simulink model "main_sim"  (Simulink 7.2)
settings: Solver=ode2  SolverMode=SingleTasking  StartTime=0.0  StopTime=tsim_max  FixedStep=dtsim  RelTol=1e-3
StopFcn:
  | %mkplt
undefined symbols (not defined in the file): aero_surf_qbar_off, aero_surf_qbar_on, assertion_time, att_type, att_type_numbers, bb_ellipsoid, bb_params, compute_all_rate_cols, compute_all_vel_cols, constants, cosA, DiscIntNeverNeededParam, dtsim, E_rwy, eow_boundary, full_surf_llim, full_surf_ulim, gain_set, gain_var_struct, MACH, MACH_att_fb, MACH_gain_mat, MACH_mass_IC, MACH_pos_IC, MACH_pqr_Bmat_IC, MACH_pqr_IC, MACH_pqr_u_IC, MACH_quat_IC, MACH_throttle_IC, MACH_U_nom_IC, MACH_vel_Bmat_IC, MACH_vel_cvdnom_IC, MACH_vel_IC, MACH_vel_uold_IC, max_LOS_rate, modes, N_rwy, pos, rcs_cvddes_thresh, reset_camcmd_on_entry, sinA, target_pos_IC, target_range_blind, target_range_detect, target_range_homing, target_vel_IC, trac_params, u_llim, u_ulim, use_auto_att_type, use_eow_as_iv, use_nav, use_pos_fltpath_lim, use_throt_estimate, use_variable_mass, use_wind_est, vel, vel_cmd_ramp_time, x_trac_IC
libraries: simulink x32, mach_lib x26, utility_lib x24, model_lib x15, simulink_need_slupdate x8, models x6
(part 4 of 5)

== system main_sim/claw_main/input processing/set control parameters/accel submode setup ==
  signal_bus : Inport  OutDataType=sfix(16)  OutScaling=2^0
  Bus Selector1 : BusSelector  OutputSignals=mode_sw.enable_homing_sw,mode_sw.accel_submode,mode_sw.CLAW_mode
  Constant1 : Constant  Value=3  OutDataType=sfix(16)  OutScaling=2^0
  Constant2 : Constant  Value=0  OutDataType=sfix(16)  OutScaling=2^0
  Merge1 : Merge  Inputs=3  InitialOutput=zeros(3,1)
  Merge2 : Merge  Inputs=3  InitialOutput=zeros(3,1)
  NED_dd/vchigam_dot : Subsystem  TreatAsAtomicUnit=on
  Switch : Switch  Threshold=0.5
  Switch Case : SwitchCase  CaseConditions={[1 2],3}
  Switch1 : Switch  Threshold=0.5  InputSameDT=on
  homing : Subsystem  TreatAsAtomicUnit=on
  normal vel desdyn : Subsystem  TreatAsAtomicUnit=on
  accel_cmd_sw : Outport  OutDataType=sfix(16)  OutScaling=2^0
  accel_cmd : Outport  Port=2  OutDataType=sfix(16)  OutScaling=2^0
  wires:
  Constant1/1 -> Switch/1
  Bus Selector1/1 -> Switch/2  "<enable_homing_sw>"
  Bus Selector1/2 -> Switch/3  "<accel_submode>"
  Switch/1 -> Switch1/1
  Switch1/1 -> Switch Case/1, NED_dd/vchigam_dot/1(case)
  Switch Case/1 -> NED_dd/vchigam_dot/Action
  Switch Case/2 -> homing/Action
  Switch Case/3 -> normal vel desdyn/Action
  Merge1/1 -> accel_cmd/1
  Merge2/1 -> accel_cmd_sw/1
  NED_dd/vchigam_dot/1(accel_cmd_sw) -> Merge2/1
  normal vel desdyn/2(accel_cmd) -> Merge1/3
  NED_dd/vchigam_dot/2(accel_cmd) -> Merge1/1
  homing/2(accel_cmd) -> Merge1/2
  homing/1(accel_cmd_sw) -> Merge2/2
  normal vel desdyn/1(accel_cmd_sw) -> Merge2/3
  Bus Selector1/3 -> Switch1/2  "<CLAW_mode>"
  Constant2/1 -> Switch1/3
  signal_bus/1 -> Bus Selector1/1, NED_dd/vchigam_dot/2(signal_bus), homing/1(signal_bus)

== system main_sim/claw_main/input processing/set control parameters/modify MACH_att_Kf ==
  gain_bus_in : Inport  OutDataType=sfix(16)  OutScaling=2^0
  signal_bus : Inport  Port=2  OutDataType=sfix(16)  OutScaling=2^0
  Bus Assignment : BusAssignment  AssignedSignals=MACH_att_Kf
  Bus Selector : BusSelector  OutputSignals=mode_sw.att_type
  Bus Selector1 : BusSelector  OutputSignals=MACH_att_Kf
  Compare To Constant : simulink/Logic and Bit Operations/Compare To Constant  SystemSampleTime=-1  relop=>=  const=att_type.mba_bank  LogicOutDataTypeMode=boolean  ZeroCross=off
  Constant : Constant  Value=MACH_att_fb  OutDataType=sfix(16)  OutScaling=2^0
  Logical Operator : Logic  AllPortsSameDT=off
  Logical Operator1 : Logic  Operator=OR  AllPortsSameDT=off  OutDataTypeMode=boolean  OutDataTypeStr=boolean
  Logical Operator2 : Logic  Operator=NOT  AllPortsSameDT=off  OutDataTypeMode=boolean  OutDataTypeStr=boolean
  Logical Operator3 : Logic  AllPortsSameDT=off  OutDataTypeMode=boolean  OutDataTypeStr=boolean
  gain_bus : Outport  OutDataType=sfix(16)  OutScaling=2^0
  wires:
  Bus Selector1/1 -> Logical Operator/1  "<MACH_att_Kf>"
  Constant/1 -> Logical Operator2/1, Logical Operator3/1
  Logical Operator2/1 -> Logical Operator1/1
  gain_bus_in/1 -> Bus Assignment/1, Bus Selector1/1
  signal_bus/1 -> Bus Selector/1
  Bus Selector/1 -> Compare To Constant/1  "<att_type>"
  Logical Operator3/1 -> Logical Operator1/2
  Compare To Constant/1 -> Logical Operator3/2
  Logical Operator1/1 -> Logical Operator/2
  Logical Operator/1 -> Bus Assignment/2
  Bus Assignment/1 -> gain_bus/1

== system main_sim/claw_main/input processing/set control parameters/select gains ==
  note: Note: Current variable gain structure will use gain_set = 1
      | if it exists, when enable_bb is true, otherwise gain_set = 0
      | (which is the global or selected default)
  enable_bb : Inport  OutDataType=sfix(16)  OutScaling=2^0
  gain_set_in : Inport  Port=2  OutDataType=sfix(16)  OutScaling=2^0
  Constant2 : Constant  Value=MACH_gain_mat  OutDataType=sfix(16)  OutScaling=2^0
  MinMax : MinMax  Inputs=2  OutDataType=sfix(16)  OutScaling=2^0
  Product : Product  Inputs=*/  OutDataType=sfix(16)  OutScaling=2^0  RndMeth=Zero
  Reshape : Reshape
  Switch : Switch
  Width1 : Width
  Width2 : Width
  mux to bus : Subsystem  mask{var_struct=gain_var_struct}
      mask prompts: var_struct "var struct"
      mask init:
      | if(~isstruct(var_struct) || length(var_struct) == 0 || ~isfield(var_struct,'name') || ~isfield(var_struct,'size'))
      |     error('var struct must be at least size 1, and must have the ''name'' and ''size'' fields defined.');
      | end
      | 
      | var_name = {var_struct.name};
      | var_size = prod(vertcat(var_struct.size),2);
      | nvar = length(var_name);
      | 
      | % remove old lines
      | nvar_old = length(get_param([gcb '/Demux'],'Outputs'));
      | for i = 1:nvar_old
      |     try
      |         delete_line(gcb,['Demux/' num2str(i)] ,['Bus Creator/' num2str(i)])
      |     end
      | end
      | 
      | set_param([gcb '/Demux'],'Outputs',mat2str(var_size));
      | set_param([gcb '/Bus Creator'],'Inputs',num2str(nvar));
      | port_handle = getfield(get_param([gcb '/Demux'],'PortHandles'),'Outport');
      | for i = 1:nvar
      |     try
      |         add_line(gcb,['Demux/' num2str(i)] ,['Bus Creator/' num2str(i)])
      |     end
      |     set(port_handle(i),'Name',var_name{i});
      | end
  select gain set : Selector  NumberOfDimensions=2  IndexMode=Zero-based  InputPortWidth=3  IndexOptions=Index vector (port),Select all  Indices=gain_set,-1  OutputSizes=1
  gain_set : Outport  OutDataType=sfix(16)  OutScaling=2^0
  gain_bus : Outport  Port=2  OutDataType=sfix(16)  OutScaling=2^0
  wires:
  Constant2/1 -> select gain set/1, Width2/1
  select gain set/1 -> Reshape/1
  Reshape/1 -> mux to bus/1(mux_in), Width1/1
  MinMax/1 -> gain_set/1, select gain set/2
  enable_bb/1 -> Switch/3
  mux to bus/1(bus_out) -> gain_bus/1
  Width2/1 -> Product/1
  Width1/1 -> Product/2
  gain_set_in/1 -> Switch/1, Switch/2
  Switch/1 -> MinMax/1
  Product/1 -> MinMax/2

== system main_sim/claw_main/input processing/set control parameters/set att desdyn params ==
  gain_bus : Inport  OutDataType=sfix(16)  OutScaling=2^0
  Bus Creator : BusCreator  Inputs=7
  Bus Selector : BusSelector  OutputSignals=MACH_att_Kb,MACH_att_Ki,MACH_att_Kaw,MACH_att_Kf
  Constant1 : Constant  Value=zeros(1,4)  OutDataType=sfix(16)  OutScaling=2^0
  Constant6 : Constant  Value=MACH_quat_IC  OutDataType=sfix(16)  OutScaling=2^0
  Signal Specification : SignalSpecification  OutDataType=sfix(16)  OutScaling=2^0
  Signal Specification1 : SignalSpecification  OutDataType=sfix(16)  OutScaling=2^0
  Signal Specification2 : SignalSpecification  OutDataType=sfix(16)  OutScaling=2^0
  compute dependent gains : mach_lib/compute dependent gains  SystemSampleTime=-1
  params : Outport  OutDataType=sfix(16)  OutScaling=2^0
  wires:
  compute dependent gains/4 -> Bus Creator/6  "x0"
  Bus Selector/3 -> compute dependent gains/3  "<MACH_att_Kaw>"
  compute dependent gains/2 -> Bus Creator/4  "ki_trim"
  compute dependent gains/1 -> Bus Creator/3  "kc"
  Bus Creator/1 -> params/1
  Bus Selector/1 -> Signal Specification/1  "<MACH_att_Kb>"
  Bus Selector/2 -> Signal Specification1/1  "<MACH_att_Ki>"
  compute dependent gains/3 -> Bus Creator/5  "kaw"
  Bus Selector/4 -> Signal Specification2/1, compute dependent gains/4  "<MACH_att_Kf>"
  gain_bus/1 -> Bus Selector/1
  Signal Specification/1 -> Bus Creator/1, compute dependent gains/2  "kb"
  Signal Specification1/1 -> Bus Creator/2, compute dependent gains/1  "ki"
  Signal Specification2/1 -> Bus Creator/7  "kf"
  Constant6/1 -> compute dependent gains/5
  Constant1/1 -> compute dependent gains/6

== system main_sim/claw_main/input processing/set control parameters/set pos desdyn params ==
  gain_bus : Inport  OutDataType=sfix(16)  OutScaling=2^0
  Bus Creator : BusCreator  Inputs=7
  Bus Selector : BusSelector  OutputSignals=MACH_pos_Kb,MACH_pos_Ki,MACH_pos_Kaw,MACH_pos_Kf
  Constant3 : Constant  Value=MACH_vel_IC  OutDataType=sfix(16)  OutScaling=2^0
  Constant6 : Constant  Value=MACH_pos_IC  OutDataType=sfix(16)  OutScaling=2^0
  Signal Specification : SignalSpecification  OutDataType=sfix(16)  OutScaling=2^0
  Signal Specification1 : SignalSpecification  OutDataType=sfix(16)  OutScaling=2^0
  Signal Specification2 : SignalSpecification  OutDataType=sfix(16)  OutScaling=2^0
  compute dependent gains : mach_lib/compute dependent gains  SystemSampleTime=-1
  params : Outport  OutDataType=sfix(16)  OutScaling=2^0
  wires:
  Bus Selector/3 -> compute dependent gains/3  "<MACH_pos_Kaw>"
  compute dependent gains/2 -> Bus Creator/4  "ki_trim"
  compute dependent gains/1 -> Bus Creator/3  "kc"
  Bus Creator/1 -> params/1
  Bus Selector/1 -> Signal Specification/1  "<MACH_pos_Kb>"
  Bus Selector/2 -> Signal Specification1/1  "<MACH_pos_Ki>"
  compute dependent gains/3 -> Bus Creator/5  "kaw"
  Bus Selector/4 -> Signal Specification2/1, compute dependent gains/4  "<MACH_pos_Kf>"
  compute dependent gains/4 -> Bus Creator/6  "x0"
  gain_bus/1 -> Bus Selector/1
  Signal Specification/1 -> Bus Creator/1, compute dependent gains/2  "kb"
  Signal Specification1/1 -> compute dependent gains/1, Bus Creator/2  "ki"
  Signal Specification2/1 -> Bus Creator/7  "kf"
  Constant6/1 -> compute dependent gains/5
  Constant3/1 -> compute dependent gains/6

== system main_sim/claw_main/input processing/set control parameters/set rate desdyn params ==
  gain_bus : Inport  OutDataType=sfix(16)  OutScaling=2^0
  Bus Creator : BusCreator  Inputs=7
  Bus Selector : BusSelector  OutputSignals=MACH_pqr_Kb,MACH_pqr_Ki,MACH_pqr_Kaw,MACH_pqr_Kf
  Constant1 : Constant  Value=zeros(1,3)  OutDataType=sfix(16)  OutScaling=2^0
  Constant6 : Constant  Value=MACH_pqr_IC  OutDataType=sfix(16)  OutScaling=2^0
  Signal Specification : SignalSpecification  OutDataType=sfix(16)  OutScaling=2^0
  Signal Specification1 : SignalSpecification  OutDataType=sfix(16)  OutScaling=2^0
  Signal Specification2 : SignalSpecification  OutDataType=sfix(16)  OutScaling=2^0
  compute dependent gains : mach_lib/compute dependent gains  SystemSampleTime=-1
  params : Outport  OutDataType=sfix(16)  OutScaling=2^0
  wires:
  Bus Selector/4 -> Signal Specification2/1  "<MACH_pqr_Kf>"
  compute dependent gains/3 -> Bus Creator/5  "kaw"
  Signal Specification1/1 -> compute dependent gains/1, Bus Creator/2  "ki"
  Signal Specification/1 -> compute dependent gains/2, Bus Creator/1  "kb"
  Bus Creator/1 -> params/1
  compute dependent gains/1 -> Bus Creator/3  "kc"
  compute dependent gains/2 -> Bus Creator/4  "ki_trim"
  Bus Selector/3 -> compute dependent gains/3  "<MACH_pqr_Kaw>"
  compute dependent gains/4 -> Bus Creator/6  "x0"
  gain_bus/1 -> Bus Selector/1
  Bus Selector/1 -> Signal Specification/1  "<MACH_pqr_Kb>"
  Bus Selector/2 -> Signal Specification1/1  "<MACH_pqr_Ki>"
  Signal Specification2/1 -> Bus Creator/7, compute dependent gains/4  "kf"
  Constant6/1 -> compute dependent gains/5
  Constant1/1 -> compute dependent gains/6

== system main_sim/claw_main/input processing/set control parameters/set rate di params ==
  full_surf : Inport  OutDataType=sfix(16)  OutScaling=2^0
  aero_env_est : Inport  Port=2  OutDataType=sfix(16)  OutScaling=2^0
  Bus Creator1 : BusCreator  Inputs=7
  Bus Selector1 : BusSelector  OutputSignals=full_surf_ulim,full_surf_llim
  Bus Selector2 : BusSelector  OutputSignals=full_surf_urlim,full_surf_lrlim
  Bus Selector3 : BusSelector  OutputSignals=qbar
  Constant5 : Constant  Value=MACH.pqr_wght_cv  OutDataType=sfix(16)  OutScaling=2^0
  Relay : Relay  OnSwitchValue=aero_surf_qbar_on  OffSwitchValue=aero_surf_qbar_off  OnOutputValue=0  OffOutputValue=1  OutDataType=sfix(16)  OutScaling=2^0
  Selector{1..2,5..6} (4 alike) : Selector  InputPortWidth=MACH.num_u  IndexOptions=Index vector (dialog)  Indices=MACH.pqr_u_idx  OutputSizes=1
  fix aero surfs when low qbar : Subsystem
  limit schedule : model_lib/no limit schedule  SystemSampleTime=-1
  select u_pref : Subsystem
  rate_params : Outport  OutDataType=sfix(16)  OutScaling=2^0
  wires:
  select u_pref/2(wght_u_pref) -> Bus Creator1/6  "wght_u_pref"
  select u_pref/1(u_pref) -> Bus Creator1/5, fix aero surfs when low qbar/4(pqr_u_pref)  "u_pref"
  Bus Creator1/1 -> rate_params/1
  full_surf/1 -> Bus Selector1/1, Bus Selector2/1, select u_pref/3(full_surf)
  Selector6/1 -> limit schedule/2
  Bus Selector1/1 -> Selector5/1  "<full_surf_ulim>"
  Bus Selector1/2 -> Selector6/1  "<full_surf_llim>"
  Selector5/1 -> limit schedule/1
  aero_env_est/1 -> select u_pref/2(aero_env_est), limit schedule/3, Bus Selector3/1
  Selector1/1 -> Bus Creator1/1  "u_urlim"
  Selector2/1 -> Bus Creator1/2  "u_lrlim"
  fix aero surfs when low qbar/1(pqr_u_ulim) -> Bus Creator1/3  "u_ulim"
  fix aero surfs when low qbar/2(pqr_u_llim) -> Bus Creator1/4  "u_llim"
  limit schedule/1 -> fix aero surfs when low qbar/1(pqr_u_ulim_in)
  limit schedule/2 -> fix aero surfs when low qbar/2(pqr_u_llim_in)
  Bus Selector2/1 -> Selector1/1  "<full_surf_urlim>"
  Bus Selector2/2 -> Selector2/1  "<full_surf_lrlim>"
  Constant5/1 -> Bus Creator1/7  "wght_cv"
  Bus Selector3/1 -> Relay/1  "<qbar>"
  Relay/1 -> fix aero surfs when low qbar/3(low_qbar), select u_pref/1(low_qbar)

== system main_sim/claw_main/input processing/set control parameters/set vel desdyn params ==
  gain_bus : Inport  OutDataType=sfix(16)  OutScaling=2^0
  Bus Creator : BusCreator  Inputs=7
  Bus Selector : BusSelector  OutputSignals=MACH_vel_Kb,MACH_vel_Ki,MACH_vel_Kaw,MACH_vel_Kf
  Constant1 : Constant  Value=MACH_vel_cvdnom_IC  OutDataType=sfix(16)  OutScaling=2^0
  Constant6 : Constant  Value=MACH_vel_IC  OutDataType=sfix(16)  OutScaling=2^0
  Signal Specification : SignalSpecification  OutDataType=sfix(16)  OutScaling=2^0
  Signal Specification1 : SignalSpecification  OutDataType=sfix(16)  OutScaling=2^0
  Signal Specification2 : SignalSpecification  OutDataType=sfix(16)  OutScaling=2^0
  compute dependent gains : mach_lib/compute dependent gains  SystemSampleTime=-1
  params : Outport  OutDataType=sfix(16)  OutScaling=2^0
  wires:
  Bus Selector/4 -> Signal Specification2/1, compute dependent gains/4  "<MACH_vel_Kf>"
  compute dependent gains/3 -> Bus Creator/5  "kaw"
  Bus Selector/2 -> Signal Specification1/1  "<MACH_vel_Ki>"
  Bus Selector/1 -> Signal Specification/1  "<MACH_vel_Kb>"
  Bus Creator/1 -> params/1
  compute dependent gains/1 -> Bus Creator/3  "kc"
  compute dependent gains/2 -> Bus Creator/4  "ki_trim"
  Bus Selector/3 -> compute dependent gains/3  "<MACH_vel_Kaw>"
  gain_bus/1 -> Bus Selector/1
  Signal Specification/1 -> Bus Creator/1, compute dependent gains/2  "kb"
  Signal Specification1/1 -> compute dependent gains/1, Bus Creator/2  "ki"
  Signal Specification2/1 -> Bus Creator/7  "kf"
  compute dependent gains/4 -> Bus Creator/6  "x0"
  Constant6/1 -> compute dependent gains/5
  Constant1/1 -> compute dependent gains/6

== system main_sim/claw_main/rate_loops/B matrix comp/cvd_def_nom ==
  x : Inport  OutDataType=sfix(16)  OutScaling=2^0
  u : Inport  Port=2  OutDataType=sfix(16)  OutScaling=2^0
  xdot : Inport  Port=3  OutDataType=sfix(16)  OutScaling=2^0
  Selector : Selector  InputPortWidth=MACH.num_x  IndexOptions=Index vector (dialog)  Indices=MACH.pqr_idx  OutputSizes=1
  Terminator : Terminator
  Terminator1 : Terminator
  cvd : Outport  OutDataType=sfix(16)  OutScaling=2^0
  wires:
  xdot/1 -> Selector/1
  Selector/1 -> cvd/1
  u/1 -> Terminator/1
  x/1 -> Terminator1/1

== system main_sim/claw_main/rate_loops/B matrix comp/cvd_def_pert ==
  x : Inport  OutDataType=sfix(16)  OutScaling=2^0
  u : Inport  Port=2  OutDataType=sfix(16)  OutScaling=2^0
  xdot : Inport  Port=3  OutDataType=sfix(16)  OutScaling=2^0
  Selector : Selector  InputPortWidth=MACH.num_x  IndexOptions=Index vector (dialog)  Indices=MACH.pqr_idx  OutputSizes=1
  Terminator : Terminator
  Terminator1 : Terminator
  cvd : Outport  OutDataType=sfix(16)  OutScaling=2^0
  wires:
  xdot/1 -> Selector/1
  Selector/1 -> cvd/1
  u/1 -> Terminator/1
  x/1 -> Terminator1/1

== system main_sim/claw_main/rate_loops/B matrix comp/pert insert ==
  X_nom : Inport  OutDataType=sfix(16)  OutScaling=2^0
  U_nom : Inport  Port=2  OutDataType=sfix(16)  OutScaling=2^0
  D_pert : Inport  Port=3  OutDataType=sfix(16)  OutScaling=2^0
  Assignment : Assignment  IndexOptions=Index vector (dialog)  Indices=MACH.pqr_u_idx  OutputSizes=[1 1]
  X_pert : Outport  OutDataType=sfix(16)  OutScaling=2^0
  U_pert : Outport  Port=2  OutDataType=sfix(16)  OutScaling=2^0
  wires:
  D_pert/1 -> Assignment/2
  Assignment/1 -> U_pert/1
  X_nom/1 -> X_pert/1
  U_nom/1 -> Assignment/1

== system main_sim/claw_main/rate_loops/B matrix comp/pert_comp ==
  col : Inport  OutDataType=sfix(16)  OutScaling=2^0
  d_nom : Inport  Port=2  OutDataType=sfix(16)  OutScaling=2^0
  params : Inport  Port=3  OutDataType=sfix(16)  OutScaling=2^0
  Bus Selector : BusSelector  OutputSignals=u_ulim,u_llim
  Constant2 : Constant  Value=diag(MACH.pqr_u_pert)  OutDataType=sfix(16)  OutScaling=2^0
  pick +/- pert : mach_lib/pick +//- pert  SystemSampleTime=-1  num_u=MACH.pqr_num_u
  d_pert : Outport  OutDataType=sfix(16)  OutScaling=2^0
  d_div : Outport  Port=2  OutDataType=sfix(16)  OutScaling=2^0
  wires:
  Constant2/1 -> pick +/- pert/5
  pick +/- pert/1 -> d_pert/1
  pick +/- pert/2 -> d_div/1  "scalar pert value"
  col/1 -> pick +/- pert/1
  d_nom/1 -> pick +/- pert/2
  Bus Selector/1 -> pick +/- pert/3  "<u_ulim>"
  params/1 -> Bus Selector/1
  Bus Selector/2 -> pick +/- pert/4  "<u_llim>"

== system main_sim/claw_main/rate_loops/allocation/RCS allocation ==
  Bmat : Inport  OutDataType=sfix(16)  OutScaling=2^0
  rcs_cmd_old : Inport  Port=2  OutDataType=sfix(16)  OutScaling=2^0
  cvd_des : Inport  Port=3  OutDataType=sfix(16)  OutScaling=2^0
  params : Inport  Port=4  OutDataType=sfix(16)  OutScaling=2^0
  Bus Selector : BusSelector  OutputSignals=wght_cv,u_ulim,u_llim
  Constant : Constant  Value=[1 1 1]  OutDataType=sfix(16)  OutScaling=2^0
  Constant1 : Constant  Value=MACH.pqr_rcs_use  OutDataType=sfix(16)  OutScaling=2^0
  Constant2 : Constant  Value=rcs_cvddes_thresh  OutDataType=sfix(16)  OutScaling=2^0
  Embedded MATLAB Function : Stateflow chart
  Sum5 : Sum  Inputs=+-|  OutDataType=sfix(16)  OutScaling=2^0  SaturateOnIntegerOverflow=on  InputSameDT=on  OutDataTypeStr=Inherit: Same as first input
  Terminator{,1..3} (4 alike) : Terminator
  rcs_cmd : Outport  OutDataType=sfix(16)  OutScaling=2^0
  cvd_extra : Outport  Port=2  OutDataType=sfix(16)  OutScaling=2^0
  wires:
  Embedded MATLAB Function/3(scale) -> Terminator3/1
  params/1 -> Bus Selector/1
  cvd_des/1 -> Sum5/2, Embedded MATLAB Function/5(cvd_des)
  Sum5/1 -> cvd_extra/1
  Bmat/1 -> Embedded MATLAB Function/1(Bmat)
  Embedded MATLAB Function/1(rcs_cmd) -> rcs_cmd/1
  Embedded MATLAB Function/2(minerr) -> Terminator2/1
  Embedded MATLAB Function/4(cvd_actual) -> Sum5/1
  rcs_cmd_old/1 -> Terminator/1
  Constant2/1 -> Embedded MATLAB Function/6(err_thresh)
  Bus Selector/3 -> Embedded MATLAB Function/4(llim)  "<u_llim>"
  Bus Selector/2 -> Embedded MATLAB Function/3(ulim)  "<u_ulim>"
  Constant1/1 -> Embedded MATLAB Function/7(rcs_use_in)
  Bus Selector/1 -> Terminator1/1  "<wght_cv>"
  Constant/1 -> Embedded MATLAB Function/2(wght_cv)

== system main_sim/claw_main/rate_loops/allocation/config_di ==
  cvd_nom : Inport  OutDataType=sfix(16)  OutScaling=2^0
  Bmat : Inport  Port=2  OutDataType=sfix(16)  OutScaling=2^0
  d_old : Inport  Port=3  OutDataType=sfix(16)  OutScaling=2^0
  d_nom : Inport  Port=4  OutDataType=sfix(16)  OutScaling=2^0
  cvd_des : Inport  Port=5  OutDataType=sfix(16)  OutScaling=2^0
  params : Inport  Port=6  OutDataType=sfix(16)  OutScaling=2^0
  di_smn : mach_lib/di_smn  SystemSampleTime=-1
  d_cmd : Outport  OutDataType=sfix(16)  OutScaling=2^0
  cvd_extra : Outport  Port=2  OutDataType=sfix(16)  OutScaling=2^0
  lambda : Outport  Port=3  OutDataType=sfix(16)  OutScaling=2^0
  solve_dat : Outport  Port=4  OutDataType=sfix(16)  OutScaling=2^0
  wires:
  cvd_nom/1 -> di_smn/1
  Bmat/1 -> di_smn/2
  d_old/1 -> di_smn/3
  d_nom/1 -> di_smn/4
  cvd_des/1 -> di_smn/5
  params/1 -> di_smn/6
  di_smn/1 -> d_cmd/1
  di_smn/2 -> cvd_extra/1
  di_smn/3 -> lambda/1
  di_smn/4 -> solve_dat/1

== system main_sim/claw_main/rate_loops/allocation/param select rcs ==
  params_all : Inport  OutDataType=sfix(16)  OutScaling=2^0
  Bus Creator1 : BusCreator  Inputs=7
  Bus Selector : BusSelector  OutputSignals=u_ulim,u_llim,u_urlim,u_lrlim,u_pref,wght_u_pref,wght_cv
  Selector{,1..5} (6 alike) : Selector  InputPortWidth=MACH.pqr_num_u  IndexOptions=Index vector (dialog)  Indices=idx  OutputSizes=1
  params : Outport  OutDataType=sfix(16)  OutScaling=2^0
  wires:
  Bus Creator1/1 -> params/1
  Bus Selector/6 -> Selector5/1  "<wght_u_pref>"
  Bus Selector/5 -> Selector4/1  "<u_pref>"
  Bus Selector/4 -> Selector3/1  "<u_lrlim>"
  Bus Selector/3 -> Selector2/1  "<u_urlim>"
  Bus Selector/2 -> Selector1/1  "<u_llim>"
  Bus Selector/1 -> Selector/1  "<u_ulim>"
  params_all/1 -> Bus Selector/1
  Selector3/1 -> Bus Creator1/4  "u_lrlim"
  Selector2/1 -> Bus Creator1/3  "u_urlim"
  Selector/1 -> Bus Creator1/1  "u_ulim"
  Selector1/1 -> Bus Creator1/2  "u_llim"
  Selector4/1 -> Bus Creator1/5  "u_pref"
  Selector5/1 -> Bus Creator1/6  "wght_u_pref"
  Bus Selector/7 -> Bus Creator1/7  "<wght_cv>"

== system main_sim/claw_main/rate_loops/allocation/param select smn ==
  params_all : Inport  OutDataType=sfix(16)  OutScaling=2^0
  Bus Creator1 : BusCreator  Inputs=7
  Bus Selector : BusSelector  OutputSignals=u_ulim,u_llim,u_urlim,u_lrlim,u_pref,wght_u_pref,wght_cv
  Selector{,1..5} (6 alike) : Selector  InputPortWidth=MACH.pqr_num_u  IndexOptions=Index vector (dialog)  Indices=idx  OutputSizes=1
  params : Outport  OutDataType=sfix(16)  OutScaling=2^0
  wires:
  Bus Selector/7 -> Bus Creator1/7  "<wght_cv>"
  Selector5/1 -> Bus Creator1/6  "wght_u_pref"
  Selector4/1 -> Bus Creator1/5  "u_pref"
  Selector1/1 -> Bus Creator1/2  "u_llim"
  Selector/1 -> Bus Creator1/1  "u_ulim"
  Selector2/1 -> Bus Creator1/3  "u_urlim"
  Selector3/1 -> Bus Creator1/4  "u_lrlim"
  params_all/1 -> Bus Selector/1
  Bus Selector/1 -> Selector/1  "<u_ulim>"
  Bus Selector/2 -> Selector1/1  "<u_llim>"
  Bus Selector/3 -> Selector2/1  "<u_urlim>"
  Bus Selector/4 -> Selector3/1  "<u_lrlim>"
  Bus Selector/5 -> Selector4/1  "<u_pref>"
  Bus Selector/6 -> Selector5/1  "<wght_u_pref>"
  Bus Creator1/1 -> params/1

== system main_sim/claw_main/rate_loops/select rate cmd/get direct cmd ==
  signal_bus : Inport  OutDataType=sfix(16)  OutScaling=2^0
  Bus Selector1 : BusSelector  OutputSignals=cmd_bus.autopilot_cmd,mode_sw.full_surf_cmd_sw,full_surf.full_surf_cmd
  Demux2 : Demux  Outputs=[ 3 1 ]
  Gain1 : Gain  Gain=MACH.throt_mixer  ParameterDataType=sfix(16)  ParameterScaling=2^0  OutDataType=sfix(16)  OutScaling=2^0
  Multiport Switch2 : MultiPortSwitch  Inputs=2  zeroidx=on
  Mux2 : Mux  Inputs=2
  throttle : Selector  InputPortWidth=MACH.num_u  IndexOptions=Index vector (dialog)  Indices=MACH.throttle_idx  OutputSizes=1
  direct_cmd : Outport  OutDataType=sfix(16)  OutScaling=2^0
  wires:
  Demux2/1 -> Mux2/1
  Demux2/2 -> Gain1/1
  Mux2/1 -> direct_cmd/1
  signal_bus/1 -> Bus Selector1/1
  Bus Selector1/1 -> Demux2/1  "<autopilot_cmd>"
  Bus Selector1/2 -> Multiport Switch2/1  "<full_surf_cmd_sw>"
  Gain1/1 -> Multiport Switch2/2
  Bus Selector1/3 -> throttle/1  "<full_surf_cmd>"
  throttle/1 -> Multiport Switch2/3
  Multiport Switch2/1 -> Mux2/2

== system main_sim/claw_main/state est/process sensors/compute dc_fltpath ==
  NEh_dot_fltpath : Inport  OutDataType=sfix(16)  OutScaling=2^0
  Gain : Gain  Gain=repmat([1 1 -1],3,1)  ParameterDataType=sfix(16)  ParameterScaling=2^0  OutDataType=sfix(16)  OutScaling=2^0
  Gain1 : Gain  Gain=[1 1 -1]  ParameterDataType=sfix(16)  ParameterScaling=2^0  OutDataType=sfix(16)  OutScaling=2^0
  Reshape : Reshape  OutputDimensionality=Customize  OutputDimensions=[3 3]
  Terminator : Terminator
  vec2dc : utility_lib/vec2dc  SystemSampleTime=-1
  dc_fltpath : Outport  OutDataType=sfix(16)  OutScaling=2^0
  wires:
  vec2dc/1 -> Reshape/1
  Reshape/1 -> Gain/1
  Gain1/1 -> vec2dc/1
  vec2dc/2 -> Terminator/1
  Gain/1 -> dc_fltpath/1
  NEh_dot_fltpath/1 -> Gain1/1

== system main_sim/claw_main/state est/process sensors/navigation complementary filter ==
  NEh nav : Inport  OutDataType=sfix(16)  OutScaling=2^0
  NEh dot : Inport  Port=2  OutDataType=sfix(16)  OutScaling=2^0
  Gain1 : Gain  Gain=MACH.K_velpos  ParameterDataType=sfix(16)  ParameterScaling=2^0  OutDataType=sfix(16)  OutScaling=2^0  SaturateOnIntegerOverflow=on  OutDataTypeStr=Inherit: Same as input  ParamDataTypeStr=Inherit: Same as input
  Sum1 : Sum  Inputs=|+-  OutDataType=sfix(16)  OutScaling=2^0  SaturateOnIntegerOverflow=on
  Sum2 : Sum  Inputs=++|  OutDataType=sfix(16)  OutScaling=2^0  SaturateOnIntegerOverflow=on  InputSameDT=on  OutDataTypeStr=Inherit: Same as first input
  integration1 : DiscreteIntegrator  SampleTime=-1  OutDataType=sfix(16)  OutScaling=2^0  ICPrevOutput=DiscIntNeverNeededParam  ICPrevScaledInput=DiscIntNeverNeededParam
  NEh_fil : Outport  OutDataType=sfix(16)  OutScaling=2^0
  wires:
  NEh dot/1 -> Sum2/1
  NEh nav/1 -> Sum1/1
  Gain1/1 -> Sum2/2
  Sum2/1 -> integration1/1
  integration1/1 -> NEh_fil/1, Sum1/2
  Sum1/1 -> Gain1/1

== system main_sim/claw_main/state est/process sensors/select e sign ==
  e in : Inport  OutDataType=sfix(16)  OutScaling=2^0
  e_past : Inport  Port=2  OutDataType=sfix(16)  OutScaling=2^0
  Dot Product : simulink/Math Operations/Dot Product  InputSameDT=on  OutDataType=sfix(16)  OutScaling=2^-10  DoSatur=off
  Gain : Gain  Gain=-1  ParameterDataType=sfix(16)  ParameterScaling=2^0  OutDataType=sfix(16)  OutScaling=2^0  SaturateOnIntegerOverflow=on  OutDataTypeStr=Inherit: Same as input  ParamDataTypeStr=Inherit: Same as input
  Switch : Switch  SaturateOnIntegerOverflow=on
  e out : Outport  OutDataType=sfix(16)  OutScaling=2^0
  wires:
  e_past/1 -> Dot Product/2
  Switch/1 -> e out/1
  Gain/1 -> Switch/3
  Dot Product/1 -> Switch/2
  e in/1 -> Gain/1, Switch/1, Dot Product/1

== system main_sim/claw_main/state est/process sensors/wait for valid nav ==
  latlonh : Inport  OutDataType=sfix(16)  OutScaling=2^0
  nav_ok : Inport  Port=2  OutDataType=sfix(16)  OutScaling=2^0
  Switch3 : Switch  Threshold=0.5  SaturateOnIntegerOverflow=on
  Unit Delay1 : UnitDelay  Orientation=left  SampleTime=-1
  LLh_0 : Outport  OutDataType=sfix(16)  OutScaling=2^0
  nav_valid : Outport  Port=2  OutDataType=sfix(16)  OutScaling=2^0
  wires:
  nav_ok/1 -> nav_valid/1, Switch3/2
  latlonh/1 -> Switch3/3
  Switch3/1 -> Unit Delay1/1, LLh_0/1
  Unit Delay1/1 -> Switch3/1

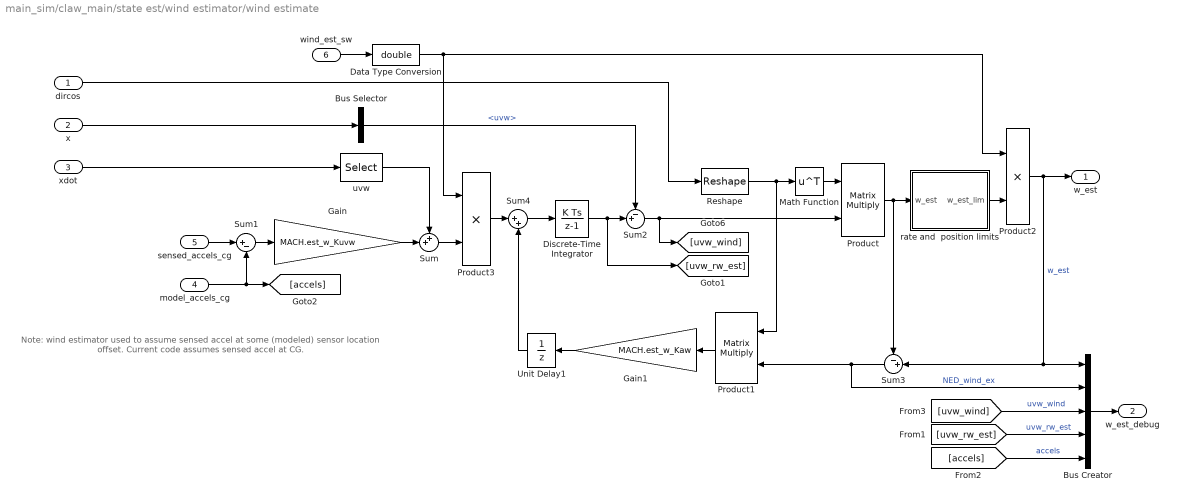
== system main_sim/claw_main/state est/wind estimator/wind estimate ==
  note: Note: wind estimator used to assume sensed accel
      | at some (modeled) sensor location offset.
      |  Current code assumes sensed accel at CG.
  dircos : Inport  OutDataType=sfix(16)  OutScaling=2^0
  x : Inport  Port=2  OutDataType=sfix(16)  OutScaling=2^0
  xdot : Inport  Port=3  OutDataType=sfix(16)  OutScaling=2^0
  model_accels_cg : Inport  Port=4  OutDataType=sfix(16)  OutScaling=2^0
  sensed_accels_cg : Inport  Port=5  OutDataType=sfix(16)  OutScaling=2^0
  wind_est_sw : Inport  Port=6  OutDataType=sfix(16)  OutScaling=2^0
  Bus Creator : BusCreator  Inputs=5
  Bus Selector : BusSelector  OutputSignals=uvw
  Data Type Conversion : DataTypeConversion  OutDataTypeMode=double  OutDataType=sfix(16)  OutScaling=2^0  OutDataTypeStr=double  SaturateOnIntegerOverflow=on  RndMeth=Zero
  Discrete-Time Integrator : DiscreteIntegrator  SampleTime=-1  OutDataType=sfix(16)  OutScaling=2^0  ICPrevOutput=DiscIntNeverNeededParam  ICPrevScaledInput=DiscIntNeverNeededParam
  Gain : Gain  Gain=MACH.est_w_Kuvw  ParameterDataType=sfix(16)  ParameterScaling=2^0  OutDataType=sfix(16)  OutScaling=2^0  SaturateOnIntegerOverflow=on  OutDataTypeStr=Inherit: Same as input  ParamDataTypeStr=Inherit: Same as input
  Gain1 : Gain  Orientation=left  Gain=MACH.est_w_Kaw  ParameterDataType=sfix(16)  ParameterScaling=2^0  OutDataType=sfix(16)  OutScaling=2^0  SaturateOnIntegerOverflow=on  OutDataTypeStr=Inherit: Same as input  ParamDataTypeStr=Inherit: Same as input
  Math Function : Math  Operator=transpose  OutDataType=sfix(16)  OutScaling=2^0  SaturateOnIntegerOverflow=on
  Product : Product  Multiplication=Matrix(*)  OutDataType=sfix(16)  OutScaling=2^0  SaturateOnIntegerOverflow=on  OutDataTypeStr=Inherit: Same as first input
  Product1 : Product  Orientation=left  Multiplication=Matrix(*)  OutDataType=sfix(16)  OutScaling=2^0  SaturateOnIntegerOverflow=on  OutDataTypeStr=Inherit: Same as first input
  Product2 : Product  OutDataType=sfix(16)  OutScaling=2^0  SaturateOnIntegerOverflow=on  OutDataTypeStr=Inherit: Same as first input
  Product3 : Product  OutDataType=sfix(16)  OutScaling=2^0  SaturateOnIntegerOverflow=on  OutDataTypeStr=Inherit: Same as first input
  Reshape : Reshape  OutputDimensionality=Customize  OutputDimensions=[3,3]
  Sum : Sum  Inputs=++|  OutDataType=sfix(16)  OutScaling=2^0  SaturateOnIntegerOverflow=on  InputSameDT=on  OutDataTypeStr=Inherit: Same as first input
  Sum1 : Sum  Inputs=|+-  OutDataType=sfix(16)  OutScaling=2^0  SaturateOnIntegerOverflow=on  InputSameDT=on  OutDataTypeStr=Inherit: Same as first input
  Sum2 : Sum  Inputs=-+|  OutDataType=sfix(16)  OutScaling=2^0  SaturateOnIntegerOverflow=on
  Sum3 : Sum  Orientation=left  Inputs=-+|  OutDataType=sfix(16)  OutScaling=2^0  SaturateOnIntegerOverflow=on
  Sum4 : Sum  Inputs=|++  OutDataType=sfix(16)  OutScaling=2^0  SaturateOnIntegerOverflow=on  InputSameDT=on  OutDataTypeStr=Inherit: Same as first input
  Unit Delay1 : UnitDelay  Orientation=left  X0=zeros(3,1)  SampleTime=-1
  rate and  position limits : Subsystem
  uvw : Selector  InputPortWidth=MACH.num_x  IndexOptions=Index vector (dialog)  Indices=MACH.uvw_idx  OutputSizes=1
  w_est : Outport  OutDataType=sfix(16)  OutScaling=2^0
  w_est_debug : Outport  Port=2  OutDataType=sfix(16)  OutScaling=2^0
  wires:
  Discrete-Time Integrator/1 -> Sum2/2, [uvw_rw_est]
  sensed_accels_cg/1 -> Sum1/1
  Sum1/1 -> Gain/1
  Sum/1 -> Product3/2
  Gain/1 -> Sum/2
  Bus Selector/1 -> Sum2/1  "<uvw>"
  dircos/1 -> Reshape/1
  Reshape/1 -> Math Function/1, Product1/1
  Product/1 -> Sum3/1, rate and  position limits/1(w_est)
  Math Function/1 -> Product/1
  Sum2/1 -> Product/2, [uvw_wind]
  Gain1/1 -> Unit Delay1/1
  xdot/1 -> uvw/1
  uvw/1 -> Sum/1
  x/1 -> Bus Selector/1
  rate and  position limits/1(w_est_lim) -> Product2/2
  Product1/1 -> Gain1/1
  Sum3/1 -> Product1/2, Bus Creator/2  "NED_wind_ex"
  Product2/1 -> w_est/1, Sum3/2, Bus Creator/1  "w_est"
  wind_est_sw/1 -> Data Type Conversion/1
  Sum4/1 -> Discrete-Time Integrator/1
  Product3/1 -> Sum4/1
  Unit Delay1/1 -> Sum4/2
  Data Type Conversion/1 -> Product2/1, Product3/1
  [uvw_wind] -> Bus Creator/3  "uvw_wind"
  [uvw_rw_est] -> Bus Creator/4  "uvw_rw_est"
  [accels] -> Bus Creator/5  "accels"
  Bus Creator/1 -> w_est_debug/1
  model_accels_cg/1 -> Sum1/2, [accels]

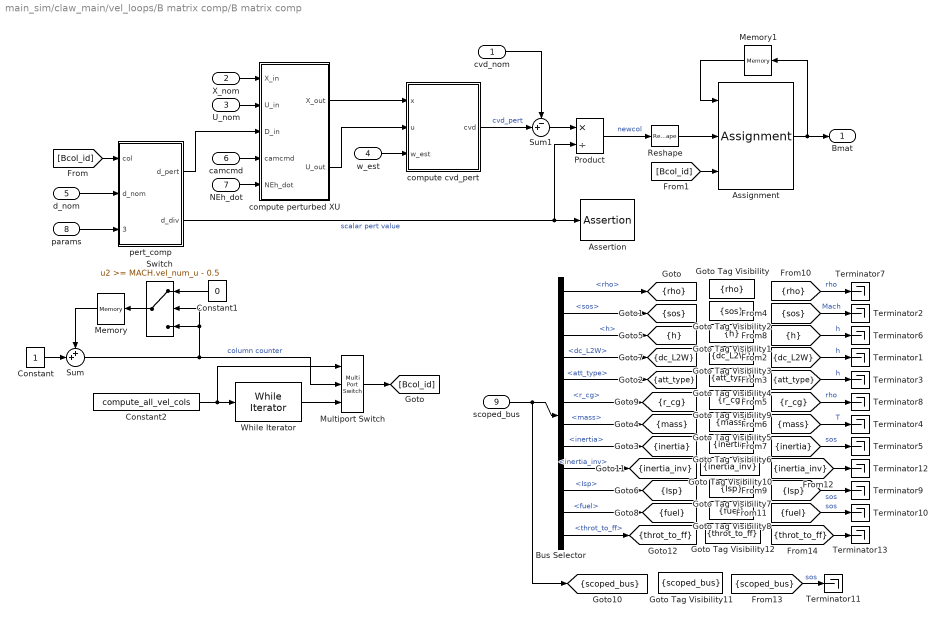
== system main_sim/claw_main/vel_loops/B matrix comp/B matrix comp ==
  cvd_nom : Inport  OutDataType=sfix(16)  OutScaling=2^0
  X_nom : Inport  Port=2  OutDataType=sfix(16)  OutScaling=2^0
  U_nom : Inport  Port=3  OutDataType=sfix(16)  OutScaling=2^0
  w_est : Inport  Port=4  OutDataType=sfix(16)  OutScaling=2^0
  d_nom : Inport  Port=5  OutDataType=sfix(16)  OutScaling=2^0
  camcmd : Inport  Port=6  OutDataType=sfix(16)  OutScaling=2^0
  NEh_dot : Inport  Port=7  OutDataType=sfix(16)  OutScaling=2^0
  params : Inport  Port=8  OutDataType=sfix(16)  OutScaling=2^0
  scoped_bus : Inport  Port=9  OutDataType=sfix(16)  OutScaling=2^0
  Assertion : Assertion  Enabled=on
  Assignment : Assignment  NumberOfDimensions=2  IndexOptions=Assign all,Index vector (port)  Indices=-1,1  OutputSizes=1,1
  Bus Selector : BusSelector  OutputSignals=atmos_env.rho,atmos_env.sos,atmos_env.h,dc_L2W,att_type,mass_props.r_cg,mass_props.mass,mass_props.inertia,mass_props.inertia_inv,mass_props.Isp,mass_props.fuel,mass_props.throt_to_ff
  Constant : Constant  OutDataType=sfix(16)  OutScaling=2^0
  Constant1 : Constant  Orientation=left  Value=0  OutDataType=sfix(16)  OutScaling=2^0
  Constant2 : Constant  Value=compute_all_vel_cols  OutDataType=sfix(16)  OutScaling=2^0
  Goto Tag Visibility : GotoTagVisibility  GotoTag=rho
  Goto Tag Visibility1 : GotoTagVisibility  GotoTag=h
  Goto Tag Visibility10 : GotoTagVisibility  GotoTag=inertia_inv
  Goto Tag Visibility11 : GotoTagVisibility  GotoTag=scoped_bus
  Goto Tag Visibility12 : GotoTagVisibility  GotoTag=throt_to_ff
  Goto Tag Visibility2 : GotoTagVisibility  GotoTag=sos
  Goto Tag Visibility3 : GotoTagVisibility  GotoTag=dc_L2W
  Goto Tag Visibility4 : GotoTagVisibility  GotoTag=att_type
  Goto Tag Visibility5 : GotoTagVisibility  GotoTag=mass
  Goto Tag Visibility6 : GotoTagVisibility  GotoTag=inertia
  Goto Tag Visibility7 : GotoTagVisibility  GotoTag=Isp
  Goto Tag Visibility8 : GotoTagVisibility  GotoTag=fuel
  Goto Tag Visibility9 : GotoTagVisibility  GotoTag=r_cg
  Memory : Memory  Orientation=left  InheritSampleTime=on
  Memory1 : Memory  Orientation=left  X0=MACH_vel_Bmat_IC  InheritSampleTime=on
  Multiport Switch : MultiPortSwitch  Inputs=2  zeroidx=on
  Product : Product  Inputs=*/  OutDataType=sfix(16)  OutScaling=2^0  SaturateOnIntegerOverflow=on  InputSameDT=on  OutDataTypeStr=Inherit: Same as first input
  Reshape : Reshape  OutputDimensionality=Column vector (2-D)
  Sum : Sum  Inputs=++|  OutDataType=sfix(16)  OutScaling=2^0  SaturateOnIntegerOverflow=on  InputSameDT=on  OutDataTypeStr=Inherit: Same as first input
  Sum1 : Sum  Inputs=-+|  OutDataType=sfix(16)  OutScaling=2^0  SaturateOnIntegerOverflow=on  InputSameDT=on  OutDataTypeStr=Inherit: Same as first input
  Switch : Switch  Orientation=left  Threshold=MACH.vel_num_u - 0.5  SaturateOnIntegerOverflow=on  InputSameDT=on
  Terminator{1..13} (13 alike) : Terminator
  While Iterator : WhileIterator  MaxIters=MACH.vel_num_u  WhileBlockType=do-while  ShowIterationPort=on
  compute cvd_pert : Subsystem
  compute perturbed XU : Subsystem
  pert_comp : Subsystem
  Bmat : Outport  OutDataType=sfix(16)  OutScaling=2^0
  tag scope: Isp=scoped, att_type=scoped, dc_L2W=scoped, fuel=scoped, h=scoped, inertia=scoped, inertia_inv=scoped, mass=scoped, r_cg=scoped, rho=scoped, scoped_bus=scoped, sos=scoped, throt_to_ff=scoped
  wires:
  U_nom/1 -> compute perturbed XU/2(U_in)
  X_nom/1 -> compute perturbed XU/1(X_in)
  Product/1 -> Reshape/1  "newcol"
  Sum1/1 -> Product/1
  [Bcol_id] -> Assignment/3
  Reshape/1 -> Assignment/2
  Assignment/1 -> Bmat/1, Memory1/1
  [Bcol_id] -> pert_comp/1(col)
  d_nom/1 -> pert_comp/2(d_nom)
  pert_comp/2(d_div) -> Product/2, Assertion/1  "scalar pert value"
  pert_comp/1(d_pert) -> compute perturbed XU/3(D_in)
  w_est/1 -> compute cvd_pert/3(w_est)
  camcmd/1 -> compute perturbed XU/4(camcmd)
  NEh_dot/1 -> compute perturbed XU/5(NEh_dot)
  compute perturbed XU/1(X_out) -> compute cvd_pert/1(x)
  params/1 -> pert_comp/3(params)
  compute perturbed XU/2(U_out) -> compute cvd_pert/2(u)
  Memory1/1 -> Assignment/1
  scoped_bus/1 -> Bus Selector/1, [scoped_bus]
  [rho] -> Terminator7/1  "rho"
  [sos] -> Terminator2/1  "Mach"
  [h] -> Terminator6/1  "h"
  Bus Selector/1 -> [rho]  "<rho>"
  Bus Selector/2 -> [sos]  "<sos>"
  Bus Selector/3 -> [h]  "<h>"
  [dc_L2W] -> Terminator1/1  "h"
  Bus Selector/4 -> [dc_L2W]  "<dc_L2W>"
  Constant2/1 -> Multiport Switch/1, While Iterator/1
  While Iterator/1 -> Multiport Switch/3
  Constant1/1 -> Switch/1
  Sum/1 -> Switch/3, Switch/2, Multiport Switch/2  "column counter"
  Switch/1 -> Memory/1
  Memory/1 -> Sum/1
  Constant/1 -> Sum/2
  Multiport Switch/1 -> [Bcol_id]
  [att_type] -> Terminator3/1  "h"
  Bus Selector/5 -> [att_type]  "<att_type>"
  [r_cg] -> Terminator8/1  "rho"
  [mass] -> Terminator4/1  "T"
  [inertia] -> Terminator5/1  "sos"
  Bus Selector/6 -> [r_cg]  "<r_cg>"
  Bus Selector/7 -> [mass]  "<mass>"
  Bus Selector/8 -> [inertia]  "<inertia>"
  [Isp] -> Terminator9/1  "sos"
  Bus Selector/10 -> [Isp]  "<Isp>"
  [fuel] -> Terminator10/1  "sos"
  Bus Selector/11 -> [fuel]  "<fuel>"
  compute cvd_pert/1(cvd) -> Sum1/2  "cvd_pert"
  cvd_nom/1 -> Sum1/1
  [inertia_inv] -> Terminator12/1
  Bus Selector/9 -> [inertia_inv]  "<inertia_inv>"
  [scoped_bus] -> Terminator11/1  "sos"
  Bus Selector/12 -> [throt_to_ff]  "<throt_to_ff>"
  [throt_to_ff] -> Terminator13/1

== system main_sim/claw_main/vel_loops/B matrix comp/compute cvd_nom ==
  note: Note: this computation of NEh accelerations
      | assumes that pqr = 0
  x : Inport  OutDataType=sfix(16)  OutScaling=2^0
  u : Inport  Port=2  OutDataType=sfix(16)  OutScaling=2^0
  w_est : Inport  Port=3  OutDataType=sfix(16)  OutScaling=2^0
  Bus Selector : BusSelector  OutputSignals=dircos
  Gain : Gain  Gain=[1 1 -1]  ParameterDataType=sfix(16)  ParameterScaling=2^0  OutDataType=sfix(16)  OutScaling=2^0  SaturateOnIntegerOverflow=on  OutDataTypeStr=Inherit: Same as input  ParamDataTypeStr=Inherit: Same as input
  Math Function : Math  Operator=transpose  OutDataType=sfix(16)  OutScaling=2^0  SaturateOnIntegerOverflow=on
  Product : Product  Multiplication=Matrix(*)  OutDataType=sfix(16)  OutScaling=2^0  SaturateOnIntegerOverflow=on  InputSameDT=on  OutDataTypeStr=Inherit: Same as first input
  Reshape : Reshape  OutputDimensionality=Customize  OutputDimensions=[3,3]
  cl model : models/gtm-obac  SystemSampleTime=-1
  uvw_dot : Selector  InputPortWidth=MACH.num_x  IndexOptions=Index vector (dialog)  Indices=MACH.uvw_idx  OutputSizes=1
  cvd : Outport  OutDataType=sfix(16)  OutScaling=2^0
  wires:
  uvw_dot/1 -> Product/2
  x/1 -> cl model/1
  Reshape/1 -> Math Function/1
  Math Function/1 -> Product/1
  Product/1 -> Gain/1
  Gain/1 -> cvd/1
  Bus Selector/1 -> Reshape/1  "<dircos>"
  u/1 -> cl model/2
  w_est/1 -> cl model/3
  cl model/1 -> uvw_dot/1
  cl model/2 -> Bus Selector/1

== system main_sim/claw_main/vel_loops/B matrix comp/compute nominal XU ==
  X_in : Inport  OutDataType=sfix(16)  OutScaling=2^0
  U_in : Inport  Port=2  OutDataType=sfix(16)  OutScaling=2^0
  D_in : Inport  Port=3  OutDataType=sfix(16)  OutScaling=2^0
  camcmd : Inport  Port=4  OutDataType=sfix(16)  OutScaling=2^0
  NEh_dot : Inport  Port=5  OutDataType=sfix(16)  OutScaling=2^0
  Assignment1 : Assignment  IndexOptions=Index vector (dialog)  Indices=MACH.throttle_idx  OutputSizes=[1 1]
  Assignment2 : Assignment  IndexOptions=Index vector (dialog)  Indices=[ MACH.quat_idx MACH.uvw_idx]  OutputSizes=[1 1]
  Demux1 : Demux  Outputs=[ 2 MACH.num_u_throt ]
  Gain : Gain  Gain=[1 1 -1]  ParameterDataType=sfix(16)  ParameterScaling=2^0  OutDataType=sfix(16)  OutScaling=2^0  SaturateOnIntegerOverflow=on  OutDataTypeStr=Inherit: Same as input  ParamDataTypeStr=Inherit: Same as input
  Mux : Mux  Inputs=[ 2 1 ]
  Mux1 : Mux  Inputs=2
  Product1 : Product  Multiplication=Matrix(*)  OutDataType=sfix(16)  OutScaling=2^0  SaturateOnIntegerOverflow=on  OutDataTypeStr=Inherit: Same as first input
  Reshape1 : Reshape  OutputDimensionality=Customize  OutputDimensions=[3,3]
  Selector1 : Selector  InputPortWidth=MACH.num_x  IndexOptions=Index vector (dialog)  Indices=MACH.quat_idx  OutputSizes=1
  att2dc : utility_lib/att2dc  SystemSampleTime=-1
  dc2e_ref : utility_lib/dc2e_ref  SystemSampleTime=-1
  X_out : Outport  OutDataType=sfix(16)  OutScaling=2^0
  U_out : Outport  Port=2  OutDataType=sfix(16)  OutScaling=2^0
  wires:
  Mux/1 -> att2dc/1
  Demux1/2 -> Assignment1/2  "throttle"
  D_in/1 -> Demux1/1
  U_in/1 -> Assignment1/1
  X_in/1 -> Assignment2/1, Selector1/1
  Assignment1/1 -> U_out/1
  camcmd/1 -> Mux/2
  Demux1/1 -> Mux/1
  NEh_dot/1 -> Gain/1
  Reshape1/1 -> Product1/1
  Assignment2/1 -> X_out/1
  att2dc/1 -> Reshape1/1, dc2e_ref/1
  dc2e_ref/1 -> Mux1/1  "e"
  Gain/1 -> Product1/2  "NED_dot"
  Selector1/1 -> dc2e_ref/2
  Product1/1 -> Mux1/2  "uvw"
  Mux1/1 -> Assignment2/2

== system main_sim/claw_main/vel_loops/convert accel_cmd to NED_dd_cmd/NED_dd cmd ==
  NEH_dd_cmd_in : Inport  OutDataType=sfix(16)  OutScaling=2^0
  Action Port : ActionPort  ActionType=case
  NEh_dd_cmd : Outport  OutDataType=sfix(16)  OutScaling=2^0  InitialOutput=zeros(3,1)
  wires:
  NEH_dd_cmd_in/1 -> NEh_dd_cmd/1

== system main_sim/claw_main/vel_loops/convert accel_cmd to NED_dd_cmd/vchigam_dot cmd ==
  vchigam_dot_cmd : Inport  OutDataType=sfix(16)  OutScaling=2^0
  NEh_d : Inport  Port=2  OutDataType=sfix(16)  OutScaling=2^0
  Action Port : ActionPort  ActionType=case
  Math Function : Math  Operator=transpose  OutDataType=sfix(16)  OutScaling=2^0  SaturateOnIntegerOverflow=on
  Product2 : Product  Multiplication=Matrix(*)  OutDataType=sfix(16)  OutScaling=2^0  RndMeth=Zero
  Reshape1 : Reshape  OutputDimensionality=Customize  OutputDimensions=[3 3]
  convert to NED_d : Gain  Gain=[1 1 -1]  ParameterDataType=sfix(16)  ParameterScaling=2^0  OutDataType=sfix(16)  OutScaling=2^0
  convert to NEh_dd : Gain  Gain=[1 1 -1]  ParameterDataType=sfix(16)  ParameterScaling=2^0  OutDataType=sfix(16)  OutScaling=2^0
  polar to cart : Subsystem
  vec2dc : utility_lib/vec2dc  SystemSampleTime=-1
  NEh_dd_cmd : Outport  OutDataType=sfix(16)  OutScaling=2^0  InitialOutput=zeros(3,1)
  wires:
  vec2dc/1 -> Reshape1/1
  Reshape1/1 -> Math Function/1
  convert to NED_d/1 -> vec2dc/1
  polar to cart/1(along_dd;cross_dd;vert_dd) -> Product2/2
  NEh_d/1 -> convert to NED_d/1
  Product2/1 -> convert to NEh_dd/1
  convert to NEh_dd/1 -> NEh_dd_cmd/1
  Math Function/1 -> Product2/1
  vchigam_dot_cmd/1 -> polar to cart/2(vchigam_dot_cmd)
  vec2dc/2 -> polar to cart/1(scaling_info)

== system main_sim/claw_main/vel_loops/set di params/att limits ==
  uvw : Inport  OutDataType=sfix(16)  OutScaling=2^0
  Bus Creator : BusCreator
  Constant : Constant  Value=MACH.vel_att_ulim  VectorParams1D=off  OutDataType=sfix(16)  OutScaling=2^0
  Constant1 : Constant  Value=MACH.vel_att_lrlim  OutDataType=sfix(16)  OutScaling=2^0
  Constant2 : Constant  Value=MACH.vel_att_urlim  OutDataType=sfix(16)  OutScaling=2^0
  Constant3 : Constant  Value=MACH.az_ulim  OutDataType=sfix(16)  OutScaling=2^0
  Constant7 : Constant  Value=MACH.vel_att_llim  VectorParams1D=off  OutDataType=sfix(16)  OutScaling=2^0
  Constant8 : Constant  Value=MACH.az_llim  OutDataType=sfix(16)  OutScaling=2^0
  Reshape1 : Reshape
  Reshape3 : Reshape
  Selector1 : Selector  NumberOfDimensions=2  InputPortWidth=3  IndexOptions=Index vector (port),Select all  Indices=1,-1  OutputSizes=1
  Selector2 : Selector  NumberOfDimensions=2  InputPortWidth=3  IndexOptions=Index vector (port),Select all  Indices=1,-1  OutputSizes=1
  velocity based angular rate llim : mach_lib/velocity based angular rate limit  SystemSampleTime=-1  q_idx=2
  velocity based angular rate ulim : mach_lib/velocity based angular rate limit  SystemSampleTime=-1  q_idx=2
  att_limits : Outport  OutDataType=sfix(16)  OutScaling=2^0
  wires:
  [att_type] -> Selector1/2, Selector2/2
  Constant/1 -> Selector1/1
  Constant7/1 -> Selector2/1
  Selector1/1 -> Reshape1/1
  Selector2/1 -> Reshape3/1
  Reshape1/1 -> Bus Creator/1  "att_ulim"
  Reshape3/1 -> Bus Creator/2  "att_llim"
  Constant2/1 -> velocity based angular rate ulim/1
  Constant8/1 -> velocity based angular rate ulim/2
  Constant1/1 -> velocity based angular rate llim/1
  Constant3/1 -> velocity based angular rate llim/2
  uvw/1 -> velocity based angular rate ulim/3, velocity based angular rate llim/3
  velocity based angular rate ulim/1 -> Bus Creator/3  "att_urlim"
  velocity based angular rate llim/1 -> Bus Creator/4  "att_lrlim"
  Bus Creator/1 -> att_limits/1

== system main_sim/claw_main/vel_loops/set di params/combine limits ==
  att_limits : Inport  OutDataType=sfix(16)  OutScaling=2^0
  throt_limits : Inport  Port=2  OutDataType=sfix(16)  OutScaling=2^0
  Bus Creator : BusCreator
  Bus Selector : BusSelector  OutputSignals=att_ulim,att_llim,att_urlim,att_lrlim
  Bus Selector1 : BusSelector  OutputSignals=throt_ulim,throt_llim,throt_urlim,throt_lrlim
  Mux{,1..3} (4 alike) : Mux  Inputs=2
  vel_u_limits : Outport  OutDataType=sfix(16)  OutScaling=2^0
  wires:
  att_limits/1 -> Bus Selector/1
  throt_limits/1 -> Bus Selector1/1
  Bus Selector/1 -> Mux/1  "<att_ulim>"
  Bus Selector/2 -> Mux1/1  "<att_llim>"
  Bus Selector/3 -> Mux2/1  "<att_urlim>"
  Bus Selector/4 -> Mux3/1  "<att_lrlim>"
  Bus Selector1/1 -> Mux/2  "<throt_ulim>"
  Bus Selector1/2 -> Mux1/2  "<throt_llim>"
  Bus Selector1/3 -> Mux2/2  "<throt_urlim>"
  Bus Selector1/4 -> Mux3/2  "<throt_lrlim>"
  Mux/1 -> Bus Creator/1  "u_ulim"
  Mux1/1 -> Bus Creator/2  "u_llim"
  Mux2/1 -> Bus Creator/3  "u_urlim"
  Mux3/1 -> Bus Creator/4  "u_lrlim"
  Bus Creator/1 -> vel_u_limits/1

== system main_sim/claw_main/vel_loops/set di params/compute dc_fltpath ==
  NEh_dot_fltpath : Inport  OutDataType=sfix(16)  OutScaling=2^0
  Gain : Gain  Gain=repmat([1 1 -1],3,1)  ParameterDataType=sfix(16)  ParameterScaling=2^0  OutDataType=sfix(16)  OutScaling=2^0
  Gain1 : Gain  Gain=[1 1 -1]  ParameterDataType=sfix(16)  ParameterScaling=2^0  OutDataType=sfix(16)  OutScaling=2^0
  Reshape : Reshape  OutputDimensionality=Customize  OutputDimensions=[3 3]
  Terminator : Terminator
  vec2dc : utility_lib/vec2dc  SystemSampleTime=-1
  dc_fltpath : Outport  OutDataType=sfix(16)  OutScaling=2^0
  wires:
  vec2dc/1 -> Reshape/1
  Reshape/1 -> Gain/1
  Gain1/1 -> vec2dc/1
  vec2dc/2 -> Terminator/1
  Gain/1 -> dc_fltpath/1
  NEh_dot_fltpath/1 -> Gain1/1

== system main_sim/claw_main/vel_loops/set di params/throttle limits ==
  full_surf : Inport  OutDataType=sfix(16)  OutScaling=2^0
  throt_old : Inport  Port=2  OutDataType=sfix(16)  OutScaling=2^0
  Bus Creator : BusCreator
  Bus Selector1 : BusSelector  OutputSignals=full_surf_ulim,full_surf_llim,full_surf_urlim,full_surf_lrlim
  Selector{1..2,5..6} (4 alike) : Selector  InputPortWidth=MACH.num_u  IndexOptions=Index vector (dialog)  Indices=MACH.throttle_idx  OutputSizes=1
  rate limit limits : mach_lib/rate limit limits  SystemSampleTime=-1  ulim=MACH.vel_throt_ulim  llim=MACH.vel_throt_llim
  throt_limits : Outport  OutDataType=sfix(16)  OutScaling=2^0
  wires:
  Bus Selector1/1 -> Selector5/1  "<full_surf_ulim>"
  Bus Selector1/2 -> Selector6/1  "<full_surf_llim>"
  full_surf/1 -> Bus Selector1/1
  throt_old/1 -> rate limit limits/1
  Selector5/1 -> rate limit limits/2
  Selector6/1 -> rate limit limits/3
  Bus Creator/1 -> throt_limits/1
  rate limit limits/1 -> Bus Creator/1  "throt_ulim"
  rate limit limits/2 -> Bus Creator/2  "throt_llim"
  Bus Selector1/3 -> Selector1/1  "<full_surf_urlim>"
  Bus Selector1/4 -> Selector2/1  "<full_surf_lrlim>"
  Selector1/1 -> rate limit limits/4, Bus Creator/3  "throt_urlim"
  Selector2/1 -> rate limit limits/5, Bus Creator/4  "throt_lrlim"

== system main_sim/vehicle_model/target/seeker model/seeker model/cart to polar ==
  note: Avoid division by zero when
      | all errors are exactly zero
  scaling info : Inport  OutDataType=sfix(16)  OutScaling=2^0
  cross_d;vert_d : Inport  Port=2  OutDataType=sfix(16)  OutScaling=2^0
  Abs : Abs
  Bus Selector : BusSelector  OutputSignals=Rground,Rslant
  Constant : Constant  Value=0.0001  OutDataType=sfix(16)  OutScaling=2^0
  Gain1 : Gain  Gain=1./max_LOS_rate  ParameterDataType=sfix(16)  ParameterScaling=2^0  OutDataType=sfix(16)  OutScaling=2^0
  Gain2 : Gain  Gain=[1 -1]  ParameterDataType=sfix(16)  ParameterScaling=2^0  OutDataType=sfix(16)  OutScaling=2^0
  MinMax : MinMax  Function=max  Inputs=3  OutDataType=sfix(16)  OutScaling=2^0
  Mux : Mux  Inputs=2
  Product : Product  Inputs=*/  OutDataType=sfix(16)  OutScaling=2^0  RndMeth=Zero
  LOS_rate : Outport  OutDataType=sfix(16)  OutScaling=2^0
  wires:
  Mux/1 -> MinMax/2
  Gain1/1 -> MinMax/1
  Gain2/1 -> Product/2
  MinMax/1 -> Gain2/1
  Abs/1 -> Gain1/1
  Product/1 -> LOS_rate/1
  cross_d;vert_d/1 -> Product/1, Abs/1
  scaling info/1 -> Bus Selector/1
  Bus Selector/1 -> Mux/1  "<Rground>"
  Bus Selector/2 -> Mux/2  "<Rslant>"
  Constant/1 -> MinMax/3
